simulink model "SB2_mfcn_done"  (R2024b)
settings: Solver=FixedStepDiscrete  StartTime=0.0  StopTime=1  FixedStep=0.05  RelTol=1e-3
settings Model: Creator=admin  LastModifiedBy=admin

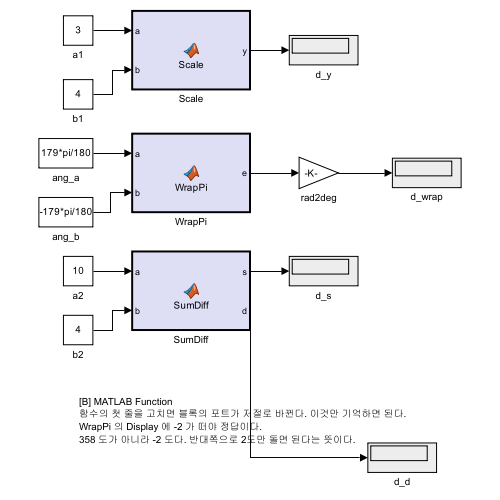
[thumbnail: Simulink's stored preview of the top-level diagram]
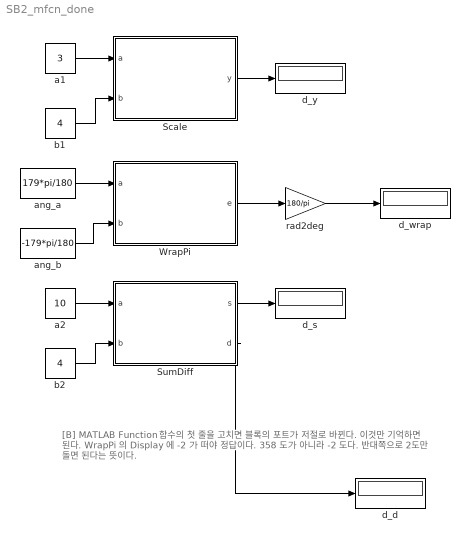
== system SB2_mfcn_done ==
  note: [B] MATLAB Function
      | 함수의 첫 줄을 고치면 블록의 포트가 저절로 바뀐다. 이것만 기억하면 된다.
      | WrapPi 의 Display 에 -2 가 떠야 정답이다.
      | 358 도가 아니라 -2 도다. 반대쪽으로 2도만 돌면 된다는 뜻이다.
  Scale : MATLAB Function  TreatAsAtomicUnit=on
  SumDiff : MATLAB Function  TreatAsAtomicUnit=on
  WrapPi : MATLAB Function  TreatAsAtomicUnit=on
  a1 : Constant  Value=3
  a2 : Constant  Value=10
  ang_a : Constant  Value=179*pi/180
  ang_b : Constant  Value=-179*pi/180
  b1 : Constant  Value=4
  b2 : Constant  Value=4
  d_d : Display
  d_s : Display
  d_wrap : Display
  d_y : Display
  rad2deg : Gain  Gain=180/pi
  wires:
  a1/1 -> Scale/1(a)
  b2/1 -> SumDiff/2(b)
  b1/1 -> Scale/2(b)
  ang_a/1 -> WrapPi/1(a)
  ang_b/1 -> WrapPi/2(b)
  a2/1 -> SumDiff/1(a)
  Scale/1(y) -> d_y/1
  WrapPi/1(e) -> rad2deg/1
  SumDiff/1(s) -> d_s/1
  rad2deg/1 -> d_wrap/1
  SumDiff/2(d) -> d_d/1

== matlab function SB2_mfcn_done/Scale ==
  data: a input; y output; b input
function y = Scale(a, b)
%#codegen
% 입력이 2개, 출력이 1개. 포트는 이 첫 줄을 그대로 따라간다.
y = a * b;

== matlab function SB2_mfcn_done/WrapPi ==
  data: a input; e output; b input
function e = WrapPi(a, b)
%#codegen
% 두 각도의 차이를 -pi ~ +pi 로 접어서 돌려준다.
% 그냥 빼기만 하면 179도와 -179도의 차이가 358도로 나온다.
d = a - b;
e = atan2(sin(d), cos(d));

== matlab function SB2_mfcn_done/SumDiff ==
  data: a input; s output; b input; d output
function [s, d] = SumDiff(a, b)
%#codegen
% 출력을 대괄호로 여러 개 적으면 출력 포트도 그만큼 생긴다.
s = a + b;
d = a - b;
